simulink model "flproj"  (R2021a)
settings: Solver=FixedStepAuto  StartTime=0.0  StopTime=2000  FixedStep=1  RelTol=1e-3
libraries: fuzblock x4
settings Model: Creator=Aleksa  LastModifiedBy=Aleksa

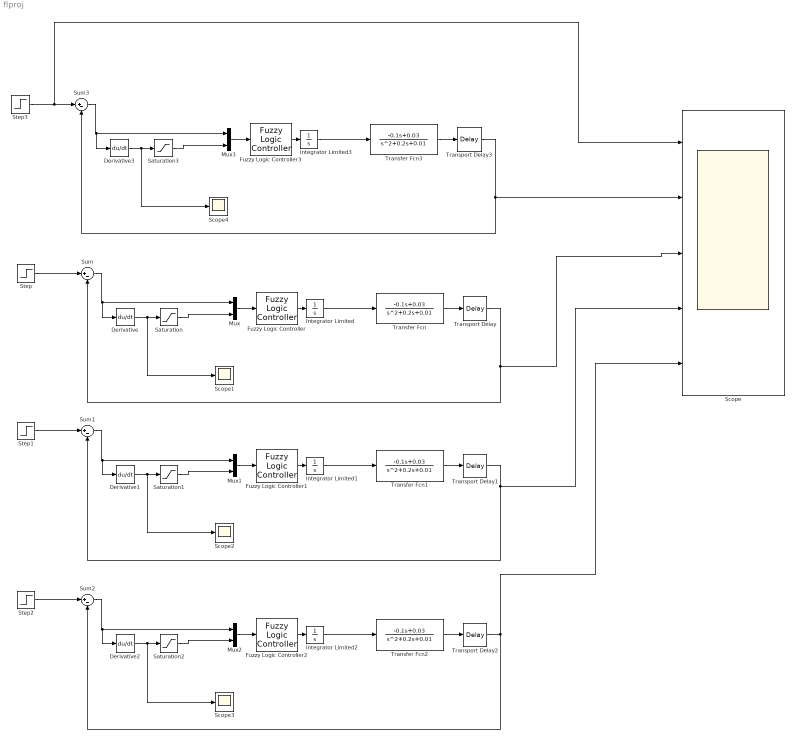
== system flproj ==
  Derivative{,1..3} (4 alike) : Derivative
  Fuzzy Logic Controller : fuzblock/Fuzzy Logic  Controller  FIS='kt125.fis'  OutputSampleNumber=101  DataType=double  FuzzifiedInputs=off  RuleFiringStrengths=off  RuleOutputs=off  AggregatedOutputs=off  SimulateUsing=Interpreted execution  OutOfRangeInputValueMessage=warning  NoRuleFiredMessage=warning  EmptyOutputFuzzySetMessage=warning
  Fuzzy Logic Controller1 : fuzblock/Fuzzy Logic  Controller  FIS='kt150.fis'  OutputSampleNumber=101  DataType=double  FuzzifiedInputs=off  RuleFiringStrengths=off  RuleOutputs=off  AggregatedOutputs=off  SimulateUsing=Interpreted execution  OutOfRangeInputValueMessage=warning  NoRuleFiredMessage=warning  EmptyOutputFuzzySetMessage=warning
  Fuzzy Logic Controller2 : fuzblock/Fuzzy Logic  Controller  FIS='kt200.fis'  OutputSampleNumber=101  DataType=double  FuzzifiedInputs=off  RuleFiringStrengths=off  RuleOutputs=off  AggregatedOutputs=off  SimulateUsing=Interpreted execution  OutOfRangeInputValueMessage=warning  NoRuleFiredMessage=warning  EmptyOutputFuzzySetMessage=warning
  Fuzzy Logic Controller3 : fuzblock/Fuzzy Logic  Controller  FIS='kt100.fis'  OutputSampleNumber=101  DataType=double  FuzzifiedInputs=off  RuleFiringStrengths=off  RuleOutputs=off  AggregatedOutputs=off  SimulateUsing=Interpreted execution  OutOfRangeInputValueMessage=warning  NoRuleFiredMessage=warning  EmptyOutputFuzzySetMessage=warning
  Integrator Limited{,1..3} (4 alike) : Integrator  LimitOutput=on  UpperSaturationLimit=1.2  LowerSaturationLimit=-1.2
  Mux{,1..3} (4 alike) : Mux  Inputs=2
  Saturation{,1..3} (4 alike) : Saturate  UpperLimit=0.1  LowerLimit=-0.1
  Scope : Scope  NumInputPorts=5
  Scope{1..4} (4 alike) : Scope
  Step{,1..3} (4 alike) : Step  Time=1000  Before=-2  After=2  SampleTime=0
  Sum{,1..3} (4 alike) : Sum  Inputs=|+-
  Transfer Fcn{,1..3} (4 alike) : TransferFcn  Numerator=[-0.1 0.03]  Denominator=[1 0.2 0.01]
  Transport Delay{,1..3} (4 alike) : TransportDelay  DelayTime=3
  wires:
  Step/1 -> Sum/1
  Transfer Fcn/1 -> Transport Delay/1
  Fuzzy Logic Controller/1 -> Integrator Limited/1
  Mux/1 -> Fuzzy Logic Controller/1
  Derivative/1 -> Scope1/1, Saturation/1
  Saturation/1 -> Mux/2
  Sum/1 -> Derivative/1, Mux/1
  Integrator Limited/1 -> Transfer Fcn/1
  Transport Delay/1 -> Scope/3, Sum/2
  Integrator Limited1/1 -> Transfer Fcn1/1
  Sum1/1 -> Mux1/1, Derivative1/1
  Saturation1/1 -> Mux1/2
  Derivative1/1 -> Saturation1/1, Scope2/1
  Mux1/1 -> Fuzzy Logic Controller1/1
  Fuzzy Logic Controller1/1 -> Integrator Limited1/1
  Transfer Fcn1/1 -> Transport Delay1/1
  Step1/1 -> Sum1/1
  Step2/1 -> Sum2/1
  Transfer Fcn2/1 -> Transport Delay2/1
  Fuzzy Logic Controller2/1 -> Integrator Limited2/1
  Mux2/1 -> Fuzzy Logic Controller2/1
  Derivative2/1 -> Scope3/1, Saturation2/1
  Saturation2/1 -> Mux2/2
  Sum2/1 -> Derivative2/1, Mux2/1
  Integrator Limited2/1 -> Transfer Fcn2/1
  Transport Delay2/1 -> Scope/5, Sum2/2
  Transport Delay3/1 -> Scope/2, Sum3/2
  Integrator Limited3/1 -> Transfer Fcn3/1
  Sum3/1 -> Mux3/1, Derivative3/1
  Saturation3/1 -> Mux3/2
  Derivative3/1 -> Saturation3/1, Scope4/1
  Mux3/1 -> Fuzzy Logic Controller3/1
  Fuzzy Logic Controller3/1 -> Integrator Limited3/1
  Transfer Fcn3/1 -> Transport Delay3/1
  Step3/1 -> Scope/1, Sum3/1
  Transport Delay1/1 -> Scope/4, Sum1/2
